simulink model "UUVModel"  (R2024b)
settings: Solver=ode4  StartTime=0.0  StopTime=100  FixedStep=0.001  RelTol=1e-3
PreLoadFcn:
  | [filepath,name,ext]  = fileparts(get_param(bdroot, 'FileName'));
  | InitFileName=[name,'_init.m'];
  | cd(filepath);
InitFcn:
  | [filepath,name,ext]  = fileparts(get_param(bdroot, 'FileName'));
  | InitFileName=[name,'_init.m'];
  | cd(filepath);
  | try
  | run(InitFileName);
  | end
values from neighbouring files (symbols this model uses):
  ESC = [ESC,ESCTmp]    [UUVModel_init.m]
  ModelParam_envAltitude = -600    [UUVModel_init.m]
  ModelParam_GPSLatLong = [ModelParam_envLatitude ModelParam_envLongitude]    [UUVModel_init.m]
  ModelParam_uavJ = [ModelParam_uavJxx,0,0;0,ModelParam_uavJyy,0;0,0,ModelParam_uavJzz]    [UUVModel_init.m]
  ModelParam_uavMass = 11.0    (= 11)    [UUVModel_init.m]
  ModelParam_uavType = int16(600)    [UUVModel_init.m]
  motor = [motor,motorTmp]    [UUVModel_init.m]
undefined symbols (not defined in the file or in its folder): Earth, ModelParam_timeSamp, UUV, WGS84
libraries: RflySimModelLab x15, aerolibtransform2 x2, aerolibatmos2 x2, sharedtransform x1, shared6dof x1, aerolibconvert2 x1, aerolibobsolete x1, aerolibasang x1, aerolibnav x1, aerolibgravity2 x1
(part 2 of 2)

== matlab function UUVModel/Force and Moment Model/UUV/浮力与重力（根据UUV） ==
  settings: updateMethod=DISCRETE
  data: DCM input; mg input; Xe input; terrainZ input; F1 output; M1 output; compensation input; height_scale_limit input; cob_origin input
%{
function [F1, M1] = fcn(DCM, mg, Xe, terrainZ, compensation, height_scale_limit, cob_origin)

F1=[0;0;0];
M1=[0;0;0];
% This is a ground model that can provides reaction force and reaction torque
mg = mg .* [1;-1;-1];
Xe = Xe .* [1;-1;-1];
terrainZ = terrainZ * -1;

length = 0.1;
% persistent z0;
% if isempty(z0)
%      z0=0;
% end
cob=Xe+cob_origin;    % 浮力作用点(earth)
z=cob(3)-terrainZ;
theta = asin(DCM(8));    % 俯仰角等于arcsin(C_32)，但是DCM为转置后的矩阵，所以这里用C_23，也就是DCM(8)

%% 计算浮力
C = compensation;    % C为补偿系数，对应ModelParam_compensation
h = height_scale_limit;    % h为浮力缩放限制高度，一般为模型高度的一半
l = length;
dz = -z;
G = -mg(3);   % 浮力为重力的反方向
% S = (h - z) / (2 * h);    % S为缩放因子
% h与z相同时，S=0，浮力消失。对应物体完全出水。
% z=0时，表示中心刚好在水面，浮力系数为1/2
% 当z=-h时，表示完全侵入水中，浮力系数为1，如果补偿系数为1，则刚好等于重力，受力平衡。

% if S > 1
%     S = 1;
% elseif S < 0
%     S = 0;
% end

h_1 = 0.5 * sqrt(h^2 + l^2) * sin(atan(h / l) + theta);
h_2 = 0.5 * sqrt(h^2 + l^2) * sin(-atan(h / l) + theta);
h_real = max(h_1, h_2);
h_out = h_real - dz;
S_1 = h * l;

if(dz >= max(abs(h_1), abs(h_2)))
    F1 = [0;0;C * G];    % 浮力
    M1 = cross(cob_origin,F1);    % 力的平移，计算力矩。 力臂 叉乘 力 等于力矩

    F1 = F1 + mg;    % 默认mg作用点在机体坐标系原点,所以直接相加
end
if(dz >= min(abs(h_1), abs(h_2)) && dz < max(abs(h_1), abs(h_2)))
    cf_out = [(l/2+l/2-h_out/sin(theta)+l/2) / 3;0;h/2+h/2+h/2-h_out/cos(theta)];
    S_out = h_out^2 / (2*sin(theta)*cos(theta));
    cf_1 = [0;0;0];
    cf_2 = cf_1 + (cf_1 - cf_out) * (S_out / (S_1 - S_out));
    
    F1 = [0;0;C * G];    % 浮力
    F_2 = F1 * (S_1 - S_out) / S_1;
    % F_2是earth坐标系，但是浮心cf_2是机体浮力坐标系的，需要转换机体坐标系再转换earth坐标系才能用于计算力矩
    cf_2 = cf_2 + cob_origin;
    cf_2 = DCM * cf_2;
    F1 = F_2;
    M1 = cross(cf_2,F1);

    F1 = F1 + mg;    % 默认mg作用点在机体坐标系原点,所以直接相加
end
if(dz < min(abs(h_1), abs(h_2)))
    if(h_1 * h_2 >= 0)
        S_1254 = h * (-h/(2 * tan(theta)) + dz/sin(theta) + l/2);
        S_345 = h^2/(2 * tan(theta));
        cf_2 = [((-l-2*h/(2*tan(theta))+2*dz/sin(theta)) / 4 * S_1254 + (-h/(2*tan(theta)) + 3*dz/sin(theta)) / 3 * S_345) / (S_1254 + S_345);...
                0;...
                ((0) / 4 * S_1254 + (-h/2) / 3 * S_345) / (S_1254 + S_345)];
        
        F1 = [0;0;C * G];    % 浮力
        F_2 = F1 * (S_1254 + S_345) / S_1;
        % F_2是earth坐标系，但是浮心cf_2是机体浮力坐标系的，需要转换机体坐标系再转换earth坐标系才能用于计算力矩
        cf_2 = cf_2 + cob_origin;
        cf_2 = DCM * cf_2;
        F1 = F_2;
        M1 = cross(cf_2,F1);

        F1 = F1 + mg;    % 默认mg作用点在机体坐标系原点,所以直接相加
    end
    if(h_1 * h_2 < 0)
        S_1235 = l * (h - (h_real - dz) / cos(theta));
        S_345 = l^2 * tan(theta) / 2;
        cf_2 = [((0) / 4 * S_1235 + (-l / 2) / 3 * S_345) / (S_1235 + S_345);...
                0;...
                ((-2 * (h_real - dz) / cos(theta)) / 4 * S_1235 + (3*h/2 - 3 * (h_real - dz) / cos(theta) + l * tan(theta)) / 3 * S_345) / (S_1235 + S_345)];
        
        F1 = [0;0;C * G];    % 浮力
        F_2 = F1 * (S_1235 + S_345) / S_1;
        % F_2是earth坐标系，但是浮心cf_2是机体浮力坐标系的，需要转换机体坐标系再转换earth坐标系才能用于计算力矩
        cf_2 = cf_2 + cob_origin;
        cf_2 = DCM * cf_2;
        F1 = F_2;
        M1 = cross(cf_2,F1);

        F1 = F1 + mg;    % 默认mg作用点在机体坐标系原点,所以直接相加
    end
end
if(dz > -max(abs(h_1), abs(h_2)) && dz <= -min(abs(h_1), abs(h_2)))
    S_123 = (h_real + dz)^2 / (2 * sin(theta) * cos(theta));
    cf_2 = [(-3 * l / 2 + (h_real + dz) / sin(theta)) / 3;...
            0;...
            (-3 * h / 2 + (h_real + dz) / cos(theta)) / 3];
    
    F1 = [0;0;C * G];    % 浮力
    F_2 = F1 * S_123 / S_1;
    % F_2是earth坐标系，但是浮心cf_2是机体浮力坐标系的，需要转换机体坐标系再转换earth坐标系才能用于计算力矩
    cf_2 = cf_2 + cob_origin;
    cf_2 = DCM * cf_2;
    F1 = F_2;
    M1 = cross(cf_2,F1);

    F1 = F1 + mg;    % 默认mg作用点在机体坐标系原点,所以直接相加
end
if(dz <= -max(abs(h_1), abs(h_2)))
    F1 = [0;0;0];
    M1 = [0;0;0];
    
    F1 = F1 + mg;    % 默认mg作用点在机体坐标系原点,所以直接相加
end
%}

%{
function [F1, M1] = fcn(DCM, mg, Xe, terrainZ, compensation, height_scale_limit, cob_origin)

F1 = [0;0;0];
M1 = [0;0;0];

% === 坐标系与符号处理（保持与你一致）===
mg = mg .* [1;-1;-1];
Xe = Xe .* [1;-1;-1];
terrainZ = terrainZ * -1;

% === 几何与物理参数 ===
length = 0.1;                     % 特征长度（你原代码中使用）
h = height_scale_limit;           % 高度半长（假设 hull 为 h x l 矩形截面）
l = length;                       % 宽度半长
g = 9.81;                         % 重力加速度
m = norm(mg) / g;                 % 质量（从 mg 推出）
V_total = 2*h * 2*l * 1.0;        % 假设单位深度（或等效体积），可标定
% 注意：若 BlueROV2 为三维体，V_total 应为实际排水体积（如 0.015 m³）
% 但此处保持与你原逻辑一致：S_1 = h*l 是截面积，故 V_total = S_1 * depth_scale
% 我们令 depth_scale = 1，因此 V_total = h * l;

% === 浮心与深度 ===
cob = Xe + cob_origin;            % 浮心在地球系（初始假设）
z = cob(3) - terrainZ;            % 浮心相对于水面的深度（正值：在水下）
dz = -z;                          % 你原代码中的 dz = -z

% === 姿态角 ===
theta = asin(DCM(8));             % 俯仰角（弧度）

% === 水密度模型（高保真关键1：深度依赖）===
% 使用简化线性模型：每100米密度增加0.2%（典型海水）
rho0 = 1025;                      % 表层海水密度 (kg/m³)
z_abs = max(0, -z);               % 深度（水面以下为正）
rho_water = rho0 * (1 + 2e-6 * z_abs * 100); % ≈ +0.02% per meter → +2% per 100m

% === 重力（始终作用于质心，假设质心在机体原点）===
F_grav = mg;                      % 已含方向，单位：N
cog_earth = Xe;                   % 质心在地球系（假设机体原点为COG）

% === 初始化浮力 ===
F_buoy = [0;0;0];
cob_earth = cob;                  % 初始浮心（后续会根据浸没状态更新）

% === 几何辅助量 ===
h_1 = 0.5 * sqrt(h^2 + l^2) * sin(atan(h / l) + theta);
h_2 = 0.5 * sqrt(h^2 + l^2) * sin(-atan(h / l) + theta);
h_real = max(h_1, h_2);
S_1 = h * l;                      % 总截面积（对应 V_total = S_1 * 1）

% === 分段计算浮力与浮心 ===
if dz >= max(abs(h_1), abs(h_2))
    % 完全浸没
    V_disp = V_total;
    cob_body = cob_origin;        % 浮心在机体坐标系（完全对称）
    F_buoy = [0; 0; rho_water * g * V_disp * compensation];
    
elseif dz >= min(abs(h_1), abs(h_2)) && dz < max(abs(h_1), abs(h_2))
    % 部分浸没：上边缘出水
    h_out = h_real - dz;
    S_out = h_out^2 / (2 * sin(theta) * cos(theta));
    S_disp = S_1 - S_out;
    V_disp = S_disp;              % 假设单位深度
    
    % 计算部分浸没浮心（简化：用几何形心）
    cf_out = [(l/2 + l/2 - h_out/sin(theta) + l/2) / 3; 0; h/2 + h/2 + h/2 - h_out/cos(theta)];
    cf_2 = cf_out + (cf_out) * (S_out / (S_1 - S_out + eps)); % 避免除零
    cob_body = -cf_2;             % 注意方向（根据你原逻辑调整）
    F_buoy = [0; 0; rho_water * g * V_disp * compensation];
    
elseif dz < min(abs(h_1), abs(h_2))
    if h_1 * h_2 >= 0
        % 侧边浸没
        S_1254 = h * (-h/(2 * tan(theta)) + dz/sin(theta) + l/2);
        S_345 = h^2/(2 * tan(theta));
        S_disp = S_1254 + S_345;
        V_disp = S_disp;
        
        cf_2 = [((-l - 2*h/(2*tan(theta)) + 2*dz/sin(theta)) / 4 * S_1254 + ...
                 (-h/(2*tan(theta)) + 3*dz/sin(theta)) / 3 * S_345) / (S_disp + eps); ...
                0; ...
                ((0) / 4 * S_1254 + (-h/2) / 3 * S_345) / (S_disp + eps)];
        cob_body = cf_2;
        F_buoy = [0; 0; rho_water * g * V_disp * compensation];
        
    else
        % 跨象限浸没
        S_1235 = l * (h - (h_real - dz) / cos(theta));
        S_345 = l^2 * tan(theta) / 2;
        S_disp = S_1235 + S_345;
        V_disp = S_disp;
        
        cf_2 = [((0) / 4 * S_1235 + (-l / 2) / 3 * S_345) / (S_disp + eps); ...
                0; ...
                ((-2 * (h_real - dz) / cos(theta)) / 4 * S_1235 + ...
                 (3*h/2 - 3 * (h_real - dz) / cos(theta) + l * tan(theta)) / 3 * S_345) / (S_disp + eps)];
        cob_body = cf_2;
        F_buoy = [0; 0; rho_water * g * V_disp * compensation];
    end
    
elseif dz > -max(abs(h_1), abs(h_2)) && dz <= -min(abs(h_1), abs(h_2))
    % 下边缘出水（较少见，保留你逻辑）
    S_123 = (h_real + dz)^2 / (2 * sin(theta) * cos(theta));
    S_disp = S_123;
    V_disp = S_disp;
    
    cf_2 = [(-3 * l / 2 + (h_real + dz) / sin(theta)) / 3; ...
            0; ...
            (-3 * h / 2 + (h_real + dz) / cos(theta)) / 3];
    cob_body = cf_2;
    F_buoy = [0; 0; rho_water * g * V_disp * compensation];
    
else
    % 完全出水
    V_disp = 0;
    F_buoy = [0;0;0];
    cob_body = cob_origin;
end

% === 转换浮心到地球系 ===
cob_earth = Xe + DCM * cob_body;

% === 总力：重力 + 浮力 ===
F1 = F_grav + F_buoy;

% === 总力矩：重力矩 + 浮力矩（相对于机体原点 Xe）===
M_grav = cross(cog_earth - Xe, F_grav);
M_buoy = cross(cob_earth - Xe, F_buoy);
M1 = M_grav + M_buoy;
end

%}

function [F1,M1] = fcn(DCM,mg,Xe,terrainZ,compensation,...
    height_scale_limit,cob_origin)

F1 = [0;0;0];
M1 = [0;0;0];

% === 坐标系处理（与你原逻辑一致）===
mg = mg .* [1;-1;-1];
Xe = Xe .* [1;-1;-1];
terrainZ = terrainZ * -1;

% === 几何参数 ===
length = 0.1;
h = height_scale_limit;    % 高度半长
l = length;                % 宽度半长
S_1 = h * l;               % 二维参考面积（m²）

% === 从输入 mg 推导质量与真实排水体积 ===
g = 9.81;
m = norm(mg) / g;          % 总质量（kg）
rho0 = 1025;               % 表层海水密度（kg/m³）
V_total_true = m / rho0;   % 中性浮力所需真实排水体积（m³）

% === 浮心与深度 ===
cob = Xe + cob_origin;
z = cob(3) - terrainZ;     % 浮心相对于水面的深度（正值：在水下）
dz = -z;

% === 姿态角（仅俯仰，保持二维）===
theta = asin(DCM(8));      % pitch angle

% === 水密度模型（深度依赖）===
z_abs = max(0, -z);        % 水面以下深度（m）
rho_water = rho0 * (1 + 2e-6 * z_abs * 100);  % ≈ +2% per 100m

% === 初始化 ===
F_grav = mg;               % 重力（已含方向）
cog_earth = Xe;            % 质心在地球系（假设在机体原点）
F_buoy = [0;0;0];
cob_body = cob_origin;     % 默认浮心

% === 几何辅助量 ===
h_1 = 0.5 * sqrt(h^2 + l^2) * sin(atan(h / l) + theta);
h_2 = 0.5 * sqrt(h^2 + l^2) * sin(-atan(h / l) + theta);
h_real = max(h_1, h_2);

% === 分段计算排水面积 S_disp ===
S_disp = 0;
if dz >= max(abs(h_1), abs(h_2))
    % 完全浸没
    S_disp = S_1;
    cob_body = cob_origin;
    
elseif dz >= min(abs(h_1), abs(h_2)) && dz < max(abs(h_1), abs(h_2))
    % 上边缘部分出水
    h_out = h_real - dz;
    S_out = h_out^2 / (2 * sin(theta) * cos(theta));
    S_disp = S_1 - S_out;
    
    cf_out = [(l/2 + l/2 - h_out/sin(theta) + l/2) / 3; 0; h/2 + h/2 + h/2 - h_out/cos(theta)];
    cf_2 = cf_out + (cf_out) * (S_out / (S_1 - S_out + eps));
    cob_body = -cf_2;
    
elseif dz < min(abs(h_1), abs(h_2))
    if h_1 * h_2 >= 0
        % 侧边浸没
        S_1254 = h * (-h/(2 * tan(theta)) + dz/sin(theta) + l/2);
        S_345 = h^2/(2 * tan(theta));
        S_disp = S_1254 + S_345;
        
        cf_2 = [((-l - 2*h/(2*tan(theta)) + 2*dz/sin(theta)) / 4 * S_1254 + ...
                 (-h/(2*tan(theta)) + 3*dz/sin(theta)) / 3 * S_345) / (S_disp + eps); ...
                0; ...
                ((0) / 4 * S_1254 + (-h/2) / 3 * S_345) / (S_disp + eps)];
        cob_body = cf_2;
        
    else
        % 跨象限浸没
        S_1235 = l * (h - (h_real - dz) / cos(theta));
        S_345 = l^2 * tan(theta) / 2;
        S_disp = S_1235 + S_345;
        
        cf_2 = [((0) / 4 * S_1235 + (-l / 2) / 3 * S_345) / (S_disp + eps); ...
                0; ...
                ((-2 * (h_real - dz) / cos(theta)) / 4 * S_1235 + ...
                 (3*h/2 - 3 * (h_real - dz) / cos(theta) + l * tan(theta)) / 3 * S_345) / (S_disp + eps)];
        cob_body = cf_2;
    end
    
elseif dz > -max(abs(h_1), abs(h_2)) && dz <= -min(abs(h_1), abs(h_2))
    % 下边缘出水（较少见）
    S_123 = (h_real + dz)^2 / (2 * sin(theta) * cos(theta));
    S_disp = S_123;
    
    cf_2 = [(-3 * l / 2 + (h_real + dz) / sin(theta)) / 3; ...
            0; ...
            (-3 * h / 2 + (h_real + dz) / cos(theta)) / 3];
    cob_body = cf_2;
    
else
    % 完全出水
    S_disp = 0;
    cob_body = cob_origin;
end

% === 将排水面积映射到真实排水体积 ===
if S_1 > 0
    V_disp = (S_disp / S_1) * V_total_true;
else
    V_disp = 0;
end

% === 计算浮力 ===
F_buoy = [0; 0; rho_water * g * V_disp * compensation];

% === 转换浮心到地球系 ===
cob_earth = Xe + DCM * cob_body;

% === 总力与总力矩 ===
F1 = F_grav + F_buoy;
M_grav = cross(cog_earth - Xe, F_grav);   % 实际为零（cog_earth = Xe）
M_buoy = cross(cob_earth - Xe, F_buoy);
M1 = M_grav + M_buoy;

end

== matlab function UUVModel/SensorOutput/HILGPSModel/GenCogVel ==
  data: v output; u input; cot output
function [v,cot] = Ang360(u)
v=norm(u(1:2));

if v < 1
    cot = 0;
else
    cot=atan2d(u(2),u(1));
end
 
if cot<0
    cot=cot+360;
end
